simulink model "cascade_realiz"  (R2020a)
settings: Solver=VariableStepAuto  StartTime=0.0  StopTime=10.0  RelTol=1e-3
settings Model: Creator=Shubham  LastModifiedBy=Shubham

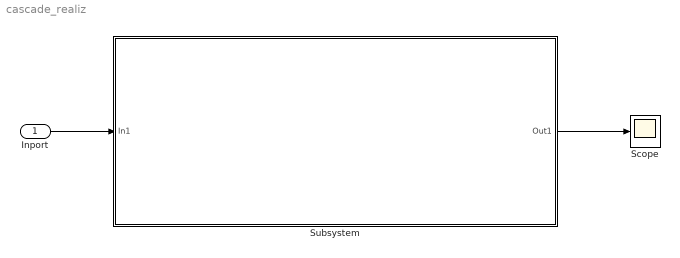
== system cascade_realiz ==
  Inport : Inport
  Scope : Scope
  Subsystem : Subsystem
  wires:
  Inport/1 -> Subsystem/1(In1)
  Subsystem/1(Out1) -> Scope/1

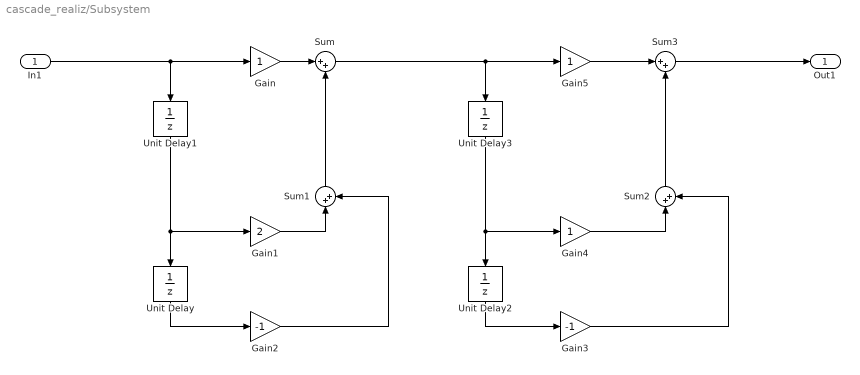
== system cascade_realiz/Subsystem ==
  In1 : Inport
  Gain : Gain
  Gain1 : Gain  Gain=2
  Gain2 : Gain  Gain=-1
  Gain3 : Gain  Gain=-1
  Gain4 : Gain
  Gain5 : Gain
  Sum{,1..3} (4 alike) : Sum  Inputs=|++
  Unit Delay{,1..3} (4 alike) : UnitDelay  SampleTime=-1  HasFrameUpgradeWarning=on
  Out1 : Outport
  wires:
  Sum/1 -> Unit Delay3/1, Gain5/1
  Sum1/1 -> Sum/2
  Unit Delay1/1 -> Unit Delay/1, Gain1/1
  Unit Delay2/1 -> Gain3/1
  Unit Delay3/1 -> Gain4/1, Unit Delay2/1
  Gain3/1 -> Sum2/2
  Unit Delay/1 -> Gain2/1
  Gain5/1 -> Sum3/1
  In1/1 -> Unit Delay1/1, Gain/1
  Gain4/1 -> Sum2/1
  Sum2/1 -> Sum3/2
  Gain/1 -> Sum/1
  Gain1/1 -> Sum1/1
  Gain2/1 -> Sum1/2
  Sum3/1 -> Out1/1
